simulink model "Full_Charge"  (R2020a)
settings: Solver=VariableStepAuto  StartTime=0.0  StopTime=45*60*60  RelTol=1e-3
values from neighbouring files (symbols this model uses):
  BlySyreON = 1    [sim_starter.m]
  CurrentChargeBlySyre = load    [sim_starter.m]
  CurrentChargeLiLille = load    [sim_starter.m]
  CurrentChargeLiStor = load    [sim_starter.m]
  CurrentChargeNiMH = load    [sim_starter.m]
  CurrentChargeSaltVand = load    [sim_starter.m]
  LiIonLilleON = 1    [sim_starter.m]
  LiIonStorON = 1    [sim_starter.m]
  NiMHON = 1    [sim_starter.m]
  SaltVandON = 1    [sim_starter.m]
  SwitchCurrentBlySyre = 1    [sim_starter.m]
  SwitchCurrentLiLille = 1    [sim_starter.m]
  SwitchCurrentLiStor = 1    [sim_starter.m]
  SwitchCurrentNiMH = 1    [sim_starter.m]
  SwitchCurrentSaltVand = 1    [sim_starter.m]
  VoltageChargeBlySyre = 0    [sim_starter.m]
  VoltageChargeLiLille = load    [sim_starter.m]
  VoltageChargeLiStor = load    [sim_starter.m]
  VoltageChargeNiMH = load    [sim_starter.m]
  VoltageChargeSaltVand = load    [sim_starter.m]
undefined symbols (not defined in the file or in its folder): Hydride, Metal, Nickel
libraries: nesl_utility x37, fl_lib x35, ee_lib x8, powerlib x7, electricdrivelib x1
(part 2 of 2)

== system Full_Charge/Opladning/SaltvandsBatteri ==
  Ah : Constant  Value=45
  Coulomb pr Ah : Constant  Value=3600
  Current Sensor1 : fl_lib/Electrical/Electrical Sensors/Current Sensor
  PS-Simulink Converter : nesl_utility/PS-Simulink Converter  PhysicalDomain=network_engine_domain  SubClassName=ps_output  LeftPortType=input  RightPortType=output  PseudoPeriodic=off  Frequencies=[]  Unit=inherit  AffineConversion=off
  PS-Simulink Converter1 : nesl_utility/PS-Simulink Converter  PhysicalDomain=network_engine_domain  SubClassName=ps_output  LeftPortType=input  RightPortType=output  PseudoPeriodic=off  Frequencies=[]  Unit=inherit  AffineConversion=off
  PS-Simulink Converter2 : nesl_utility/PS-Simulink Converter  PhysicalDomain=network_engine_domain  SubClassName=ps_output  LeftPortType=input  RightPortType=output  PseudoPeriodic=off  Frequencies=[]  Unit=inherit  AffineConversion=off
  Percent SOC : Product  Inputs=*/
  Saltvands : ee_lib/Sources/Battery  Vnom=12 V  R1=0.005 Ohm  prm_AH=2  AH=45 hr*A  V1=10.8 V  AH1=2 hr*A  prm_R2=1  R2=5000 Ohm  prm_dyn=3  Rp1=0.05 Ohm  tau1=700 s  Rp2=0.01 Ohm  tau2=55 s  Rp3=0.005 Ohm  tau3=30 s  Rp4=0.005 Ohm  tau4=30 s  Rp5=0.005 Ohm  tau5=30 s  prm_fade=2  N_fade=5000  AH_fade=36 hr*A  R1_fade=2.02 Ohm  V1_fade=10.35 V  i_specify=off  i_priority=None  i=0 A  i_nominal_specify=off  i_nominal_unit=A  i_nominal_value=1  v_specify=off  v_priority=None  v=0 V  v_nominal_specify=off  v_nominal_unit=V  v_nominal_value=1  charge_specify=on  charge_priority=High  charge=4.5 hr*A  charge_nominal_specify=off  charge_nominal_unit=hr*A  charge_nominal_value=1  num_cycles_specify=off  num_cycles_priority=High  num_cycles=20  num_cycles_nominal_specify=off  num_cycles_nominal_unit=1  num_cycles_nominal_value=1  thermal_mass=30000 J/K  Tmeas=298.15 K  Vnom_T2=12 V  R1_T2=2.2 Ohm  V1_T2=11.4 V  R2_T2=2200 Ohm  Rp1_T2=0.005 Ohm  tau1_T2=30 s  Rp2_T2=0.005 Ohm  tau2_T2=30 s  Rp3_T2=0.005 Ohm  tau3_T2=30 s  Rp4_T2=0.005 Ohm  tau4_T2=30 s  Rp5_T2=0.005 Ohm  tau5_T2=30 s  Tmeas2=273.15 K  temperature_specify=off  temperature_priority=High  temperature=298.15 K  temperature_nominal_specify=off  temperature_nominal_unit=K  temperature_nominal_value=1
      settings: LogSimulationData=on  InternalSimscapePortConfiguration="{\"Bottom\":[],\"Left\":[{\"id\":\"p\",\"label\":\"+\",\"type\":\"foundation.electrical.electrical\"},{\"id\":\"q\",\"label\":\"q\",\"type\":\"output\"}],\"Right\":[{\"id\":\"n\",\"label\":\"-\",\"type\":\"foundation.electrical.electrical\"}],\"Top\":[]}"
  Solver Configuration1 : nesl_utility/Solver Configuration  PhysicalDomain=network_engine_domain  SubClassName=solver  LeftPortType=input  RightPortType=generic  Tones=[]  Harmonics=[]  SimulateNoise=off  Profile=off  UseLocalSampling=off  EnableSwitchedLinearOptims=on  FrequencyDomain=off  UseCCode=off  RelTol=0.001  AbsTol=1e-06  MinStep=1e-09  ToWorkspace=off  RevertToSquareIcSolve=off  NumHomotopyIterations=100  PhasorMode=off  PhasorModeNumHarmonics=1  DoDC=off  ResidualTolerance=1e-09  UseLocalSolver=off  LocalSolverChoice=NE_BACKWARD_EULER_ADVANCER  LocalSolverSampleTime=0.001  DoFixedCost=off  MaxNonlinIter=3  MaxModeIter=2  LinearAlgebra=auto  EquationFormulation=NE_TIME_EF  DelaysMemoryBudget=1024  AutomaticFiltering=on  FilteringTimeConstant=0.001  PartitionStorageMethod=AS_NEEDED  PartitionMemoryBudget=1024  PartitionMethod=ROBUST
  Total Coulomb : Product  Inputs=**
  Voltage Sensor1 : fl_lib/Electrical/Electrical Sensors/Voltage Sensor
  Positiv pin : PMIOPort  Side=Right
  Negativ pin : PMIOPort  Port=2  Side=Right
  voltage : Outport
  current : Outport  Port=2
  SOC : Outport  Port=3
  wires:
  PS-Simulink Converter/1 -> current/1  "Current"
  PS-Simulink Converter1/1 -> voltage/1  "Voltage"
  Total Coulomb/1 -> Percent SOC/2
  PS-Simulink Converter2/1 -> Percent SOC/1  "Current Coulomb"
  Percent SOC/1 -> SOC/1  "State of Charge"
  Ah/1 -> Total Coulomb/1
  Coulomb pr Ah/1 -> Total Coulomb/2
  connections:
  Voltage Sensor1/RConn2 -- Saltvands/RConn1 -- Current Sensor1/RConn2
  Saltvands/LConn1 -- Positiv pin/RConn1 -- Voltage Sensor1/LConn1 -- Solver Configuration1/RConn1
  Current Sensor1/LConn1 -- Negativ pin/RConn1
  Current Sensor1/RConn1 -- PS-Simulink Converter/LConn1
  Voltage Sensor1/RConn1 -- PS-Simulink Converter1/LConn1
  Saltvands/LConn2 -- PS-Simulink Converter2/LConn1

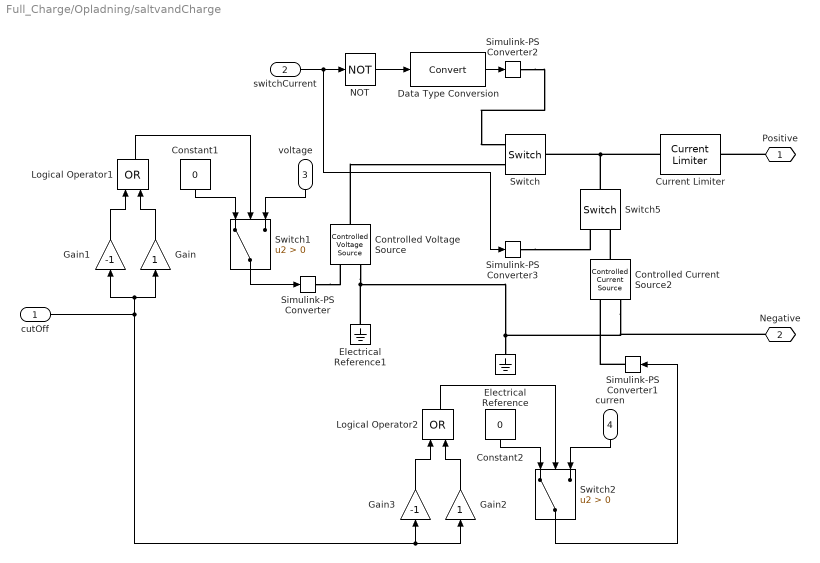
== system Full_Charge/Opladning/saltvandCharge ==
  cutOff : Inport
  switchCurrent : Inport  Port=2
  voltage : Inport  Port=3
  curren : Inport  Port=4
  Constant1 : Constant  Value=0
  Constant2 : Constant  Value=0
  Controlled Current Source2 : fl_lib/Electrical/Electrical Sources/Controlled Current Source
  Controlled Voltage Source : fl_lib/Electrical/Electrical Sources/Controlled Voltage Source
  Current Limiter : ee_lib/Semiconductors & Converters/Current Limiter  iLim=20 A  vLim=0.1 V  gLim=1e-3 1/Ohm  thermal_mass=100 J/K  initial_temperature=298.15 K
      settings: SourceProductBaseCode=PS  InternalSimscapePortConfiguration="{\"Bottom\":[],\"Left\":[{\"id\":\"p\",\"label\":\"+\",\"type\":\"foundation.electrical.electrical\"}],\"Right\":[{\"id\":\"n\",\"label\":\"-\",\"type\":\"foundation.electrical.electrical\"}],\"Top\":[]}"
  Data Type Conversion : DataTypeConversion
  Electrical Reference : fl_lib/Electrical/Electrical Elements/Electrical Reference
  Electrical Reference1 : fl_lib/Electrical/Electrical Elements/Electrical Reference
  Gain : Gain
  Gain1 : Gain  Gain=-1
  Gain2 : Gain
  Gain3 : Gain  Gain=-1
  Logical Operator1 : Logic  Operator=OR  AllPortsSameDT=off  OutDataTypeStr=boolean
  Logical Operator2 : Logic  Operator=OR  AllPortsSameDT=off  OutDataTypeStr=boolean
  NOT : Logic  Operator=NOT  IconShape=distinctive  AllPortsSameDT=off  OutDataTypeStr=boolean
  Simulink-PS Converter : nesl_utility/Simulink-PS Converter  PhysicalDomain=network_engine_domain  SubClassName=ps_input  LeftPortType=input  RightPortType=output  PseudoPeriodic=off  Frequencies=[]  NoiseDistribution=none  NoiseParameters=[]  Unit=V  AffineConversion=off  FilteringAndDerivatives=provide  SimscapeFilterOrder=1  InputFilterTimeConstant=0.001  UdotUserProvided=0
  Simulink-PS Converter1 : nesl_utility/Simulink-PS Converter  PhysicalDomain=network_engine_domain  SubClassName=ps_input  LeftPortType=input  RightPortType=output  PseudoPeriodic=off  Frequencies=[]  NoiseDistribution=none  NoiseParameters=[]  Unit=A  AffineConversion=off  FilteringAndDerivatives=provide  SimscapeFilterOrder=1  InputFilterTimeConstant=0.001  UdotUserProvided=0
  Simulink-PS Converter2 : nesl_utility/Simulink-PS Converter  PhysicalDomain=network_engine_domain  SubClassName=ps_input  LeftPortType=input  RightPortType=output  PseudoPeriodic=off  Frequencies=[]  NoiseDistribution=none  NoiseParameters=[]  Unit=V  AffineConversion=off  FilteringAndDerivatives=provide  SimscapeFilterOrder=1  InputFilterTimeConstant=0.001  UdotUserProvided=0
  Simulink-PS Converter3 : nesl_utility/Simulink-PS Converter  PhysicalDomain=network_engine_domain  SubClassName=ps_input  LeftPortType=input  RightPortType=output  PseudoPeriodic=off  Frequencies=[]  NoiseDistribution=none  NoiseParameters=[]  Unit=V  AffineConversion=off  FilteringAndDerivatives=provide  SimscapeFilterOrder=1  InputFilterTimeConstant=0.001  UdotUserProvided=0
  Switch : fl_lib/Electrical/Electrical Elements/Switch  R_closed=0.01 Ohm  G_open=1e-8 1/Ohm  Threshold=0.5  i_specify=off  i_priority=None  i=0 A  i_nominal_specify=off  i_nominal_unit=A  i_nominal_value=1  v_specify=off  v_priority=None  v=0 V  v_nominal_specify=off  v_nominal_unit=V  v_nominal_value=1
  Switch1 : Switch  Criteria=u2 > Threshold
  Switch2 : Switch  Criteria=u2 > Threshold
  Switch5 : fl_lib/Electrical/Electrical Elements/Switch  R_closed=0.01 Ohm  G_open=1e-8 1/Ohm  Threshold=0.5  i_specify=off  i_priority=None  i=0 A  i_nominal_specify=off  i_nominal_unit=A  i_nominal_value=1  v_specify=off  v_priority=None  v=0 V  v_nominal_specify=off  v_nominal_unit=V  v_nominal_value=1
  Positive : PMIOPort  Side=Left
  Negative : PMIOPort  Port=2  Side=Left
  wires:
  Constant1/1 -> Switch1/1
  Logical Operator1/1 -> Switch1/2
  Gain3/1 -> Logical Operator2/1
  Logical Operator2/1 -> Switch2/2
  Gain/1 -> Logical Operator1/2
  switchCurrent/1 -> Simulink-PS Converter3/1, NOT/1
  NOT/1 -> Data Type Conversion/1
  curren/1 -> Switch2/3
  cutOff/1 -> Gain3/1, Gain2/1, Gain1/1, Gain/1
  Gain2/1 -> Logical Operator2/2
  Gain1/1 -> Logical Operator1/1
  Switch1/1 -> Simulink-PS Converter/1
  voltage/1 -> Switch1/3
  Data Type Conversion/1 -> Simulink-PS Converter2/1
  Constant2/1 -> Switch2/1
  Switch2/1 -> Simulink-PS Converter1/1
  connections:
  Current Limiter/LConn1 -- Switch5/LConn1 -- Switch/LConn1
  Controlled Voltage Source/RConn2 -- Electrical Reference1/LConn1 -- Electrical Reference/LConn1 -- Negative/RConn1 -- Controlled Current Source2/RConn2
  Simulink-PS Converter3/RConn1 -- Switch5/RConn1
  Positive/RConn1 -- Current Limiter/RConn1
  Simulink-PS Converter/RConn1 -- Controlled Voltage Source/RConn1
  Simulink-PS Converter2/RConn1 -- Switch/RConn1
  Simulink-PS Converter1/RConn1 -- Controlled Current Source2/RConn1
  Controlled Voltage Source/LConn1 -- Switch/RConn2
  Controlled Current Source2/LConn1 -- Switch5/RConn2

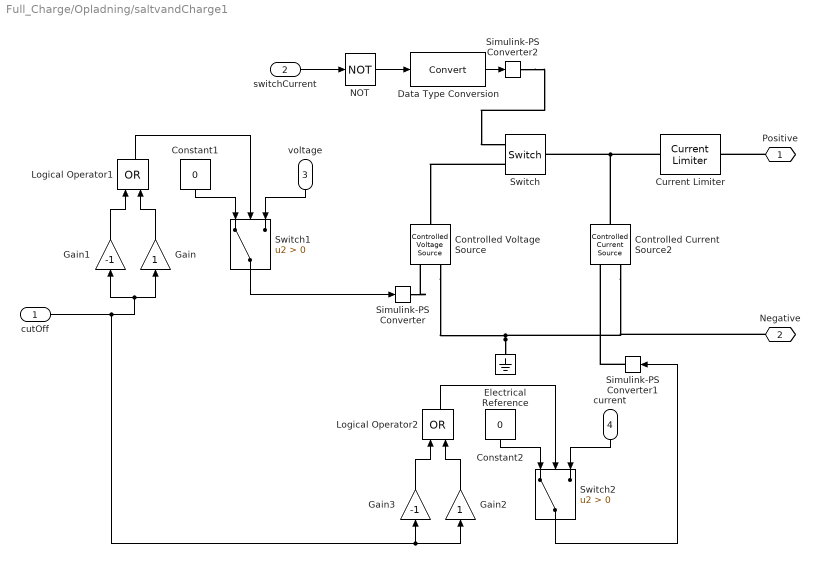
== system Full_Charge/Opladning/saltvandCharge1 ==
  cutOff : Inport
  switchCurrent : Inport  Port=2
  voltage : Inport  Port=3
  current : Inport  Port=4
  Constant1 : Constant  Value=0
  Constant2 : Constant  Value=0
  Controlled Current Source2 : fl_lib/Electrical/Electrical Sources/Controlled Current Source
  Controlled Voltage Source : fl_lib/Electrical/Electrical Sources/Controlled Voltage Source
  Current Limiter : ee_lib/Semiconductors & Converters/Current Limiter  iLim=19 A  vLim=0.1 V  gLim=1e-3 1/Ohm  thermal_mass=100 J/K  initial_temperature=298.15 K
      settings: SourceProductBaseCode=PS  InternalSimscapePortConfiguration="{\"Bottom\":[],\"Left\":[{\"id\":\"p\",\"label\":\"+\",\"type\":\"foundation.electrical.electrical\"}],\"Right\":[{\"id\":\"n\",\"label\":\"-\",\"type\":\"foundation.electrical.electrical\"}],\"Top\":[]}"
  Data Type Conversion : DataTypeConversion
  Electrical Reference : fl_lib/Electrical/Electrical Elements/Electrical Reference
  Gain : Gain
  Gain1 : Gain  Gain=-1
  Gain2 : Gain
  Gain3 : Gain  Gain=-1
  Logical Operator1 : Logic  Operator=OR  AllPortsSameDT=off  OutDataTypeStr=boolean
  Logical Operator2 : Logic  Operator=OR  AllPortsSameDT=off  OutDataTypeStr=boolean
  NOT : Logic  Operator=NOT  IconShape=distinctive  AllPortsSameDT=off  OutDataTypeStr=boolean
  Simulink-PS Converter : nesl_utility/Simulink-PS Converter  PhysicalDomain=network_engine_domain  SubClassName=ps_input  LeftPortType=input  RightPortType=output  PseudoPeriodic=off  Frequencies=[]  NoiseDistribution=none  NoiseParameters=[]  Unit=V  AffineConversion=off  FilteringAndDerivatives=provide  SimscapeFilterOrder=1  InputFilterTimeConstant=0.001  UdotUserProvided=0
  Simulink-PS Converter1 : nesl_utility/Simulink-PS Converter  PhysicalDomain=network_engine_domain  SubClassName=ps_input  LeftPortType=input  RightPortType=output  PseudoPeriodic=off  Frequencies=[]  NoiseDistribution=none  NoiseParameters=[]  Unit=A  AffineConversion=off  FilteringAndDerivatives=provide  SimscapeFilterOrder=1  InputFilterTimeConstant=0.001  UdotUserProvided=0
  Simulink-PS Converter2 : nesl_utility/Simulink-PS Converter  PhysicalDomain=network_engine_domain  SubClassName=ps_input  LeftPortType=input  RightPortType=output  PseudoPeriodic=off  Frequencies=[]  NoiseDistribution=none  NoiseParameters=[]  Unit=V  AffineConversion=off  FilteringAndDerivatives=provide  SimscapeFilterOrder=1  InputFilterTimeConstant=0.001  UdotUserProvided=0
  Switch : fl_lib/Electrical/Electrical Elements/Switch  R_closed=0.01 Ohm  G_open=1e-8 1/Ohm  Threshold=0.5  i_specify=off  i_priority=None  i=0 A  i_nominal_specify=off  i_nominal_unit=A  i_nominal_value=1  v_specify=off  v_priority=None  v=0 V  v_nominal_specify=off  v_nominal_unit=V  v_nominal_value=1
  Switch1 : Switch  Criteria=u2 > Threshold
  Switch2 : Switch  Criteria=u2 > Threshold
  Positive : PMIOPort  Side=Left
  Negative : PMIOPort  Port=2  Side=Left
  wires:
  Data Type Conversion/1 -> Simulink-PS Converter2/1
  NOT/1 -> Data Type Conversion/1
  switchCurrent/1 -> NOT/1
  voltage/1 -> Switch1/3
  Constant1/1 -> Switch1/1
  Logical Operator1/1 -> Switch1/2
  Gain1/1 -> Logical Operator1/1
  Switch1/1 -> Simulink-PS Converter/1
  Gain/1 -> Logical Operator1/2
  cutOff/1 -> Gain3/1, Gain2/1, Gain1/1, Gain/1
  Gain2/1 -> Logical Operator2/2
  current/1 -> Switch2/3
  Gain3/1 -> Logical Operator2/1
  Constant2/1 -> Switch2/1
  Logical Operator2/1 -> Switch2/2
  Switch2/1 -> Simulink-PS Converter1/1
  connections:
  Positive/RConn1 -- Current Limiter/RConn1
  Switch/RConn2 -- Controlled Voltage Source/LConn1
  Simulink-PS Converter1/RConn1 -- Controlled Current Source2/RConn1
  Simulink-PS Converter2/RConn1 -- Switch/RConn1
  Simulink-PS Converter/RConn1 -- Controlled Voltage Source/RConn1
  Electrical Reference/LConn1 -- Controlled Voltage Source/RConn2 -- Controlled Current Source2/RConn2 -- Negative/RConn1
  Current Limiter/LConn1 -- Controlled Current Source2/LConn1 -- Switch/LConn1

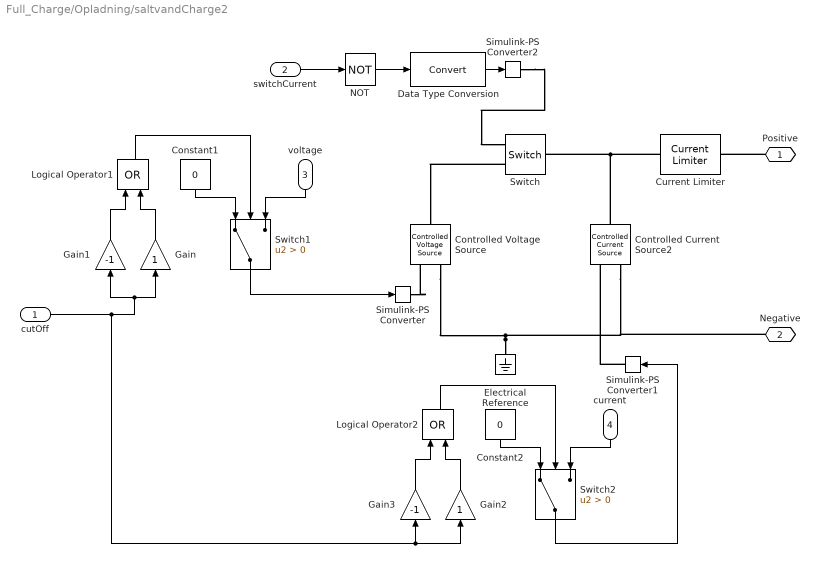
== system Full_Charge/Opladning/saltvandCharge2 ==
  cutOff : Inport
  switchCurrent : Inport  Port=2
  voltage : Inport  Port=3
  current : Inport  Port=4
  Constant1 : Constant  Value=0
  Constant2 : Constant  Value=0
  Controlled Current Source2 : fl_lib/Electrical/Electrical Sources/Controlled Current Source
  Controlled Voltage Source : fl_lib/Electrical/Electrical Sources/Controlled Voltage Source
  Current Limiter : ee_lib/Semiconductors & Converters/Current Limiter  iLim=19 A  vLim=0.1 V  gLim=1e-3 1/Ohm  thermal_mass=100 J/K  initial_temperature=298.15 K
      settings: SourceProductBaseCode=PS  InternalSimscapePortConfiguration="{\"Bottom\":[],\"Left\":[{\"id\":\"p\",\"label\":\"+\",\"type\":\"foundation.electrical.electrical\"}],\"Right\":[{\"id\":\"n\",\"label\":\"-\",\"type\":\"foundation.electrical.electrical\"}],\"Top\":[]}"
  Data Type Conversion : DataTypeConversion
  Electrical Reference : fl_lib/Electrical/Electrical Elements/Electrical Reference
  Gain : Gain
  Gain1 : Gain  Gain=-1
  Gain2 : Gain
  Gain3 : Gain  Gain=-1
  Logical Operator1 : Logic  Operator=OR  AllPortsSameDT=off  OutDataTypeStr=boolean
  Logical Operator2 : Logic  Operator=OR  AllPortsSameDT=off  OutDataTypeStr=boolean
  NOT : Logic  Operator=NOT  IconShape=distinctive  AllPortsSameDT=off  OutDataTypeStr=boolean
  Simulink-PS Converter : nesl_utility/Simulink-PS Converter  PhysicalDomain=network_engine_domain  SubClassName=ps_input  LeftPortType=input  RightPortType=output  PseudoPeriodic=off  Frequencies=[]  NoiseDistribution=none  NoiseParameters=[]  Unit=V  AffineConversion=off  FilteringAndDerivatives=provide  SimscapeFilterOrder=1  InputFilterTimeConstant=0.001  UdotUserProvided=0
  Simulink-PS Converter1 : nesl_utility/Simulink-PS Converter  PhysicalDomain=network_engine_domain  SubClassName=ps_input  LeftPortType=input  RightPortType=output  PseudoPeriodic=off  Frequencies=[]  NoiseDistribution=none  NoiseParameters=[]  Unit=A  AffineConversion=off  FilteringAndDerivatives=provide  SimscapeFilterOrder=1  InputFilterTimeConstant=0.001  UdotUserProvided=0
  Simulink-PS Converter2 : nesl_utility/Simulink-PS Converter  PhysicalDomain=network_engine_domain  SubClassName=ps_input  LeftPortType=input  RightPortType=output  PseudoPeriodic=off  Frequencies=[]  NoiseDistribution=none  NoiseParameters=[]  Unit=V  AffineConversion=off  FilteringAndDerivatives=provide  SimscapeFilterOrder=1  InputFilterTimeConstant=0.001  UdotUserProvided=0
  Switch : fl_lib/Electrical/Electrical Elements/Switch  R_closed=0.01 Ohm  G_open=1e-8 1/Ohm  Threshold=0.5  i_specify=off  i_priority=None  i=0 A  i_nominal_specify=off  i_nominal_unit=A  i_nominal_value=1  v_specify=off  v_priority=None  v=0 V  v_nominal_specify=off  v_nominal_unit=V  v_nominal_value=1
  Switch1 : Switch  Criteria=u2 > Threshold
  Switch2 : Switch  Criteria=u2 > Threshold
  Positive : PMIOPort  Side=Left
  Negative : PMIOPort  Port=2  Side=Left
  wires:
  Data Type Conversion/1 -> Simulink-PS Converter2/1
  NOT/1 -> Data Type Conversion/1
  switchCurrent/1 -> NOT/1
  voltage/1 -> Switch1/3
  Constant1/1 -> Switch1/1
  Logical Operator1/1 -> Switch1/2
  Gain1/1 -> Logical Operator1/1
  Switch1/1 -> Simulink-PS Converter/1
  Gain/1 -> Logical Operator1/2
  cutOff/1 -> Gain3/1, Gain2/1, Gain1/1, Gain/1
  Gain2/1 -> Logical Operator2/2
  current/1 -> Switch2/3
  Gain3/1 -> Logical Operator2/1
  Constant2/1 -> Switch2/1
  Logical Operator2/1 -> Switch2/2
  Switch2/1 -> Simulink-PS Converter1/1
  connections:
  Positive/RConn1 -- Current Limiter/RConn1
  Switch/RConn2 -- Controlled Voltage Source/LConn1
  Simulink-PS Converter1/RConn1 -- Controlled Current Source2/RConn1
  Simulink-PS Converter2/RConn1 -- Switch/RConn1
  Simulink-PS Converter/RConn1 -- Controlled Voltage Source/RConn1
  Electrical Reference/LConn1 -- Controlled Voltage Source/RConn2 -- Controlled Current Source2/RConn2 -- Negative/RConn1
  Current Limiter/LConn1 -- Controlled Current Source2/LConn1 -- Switch/LConn1

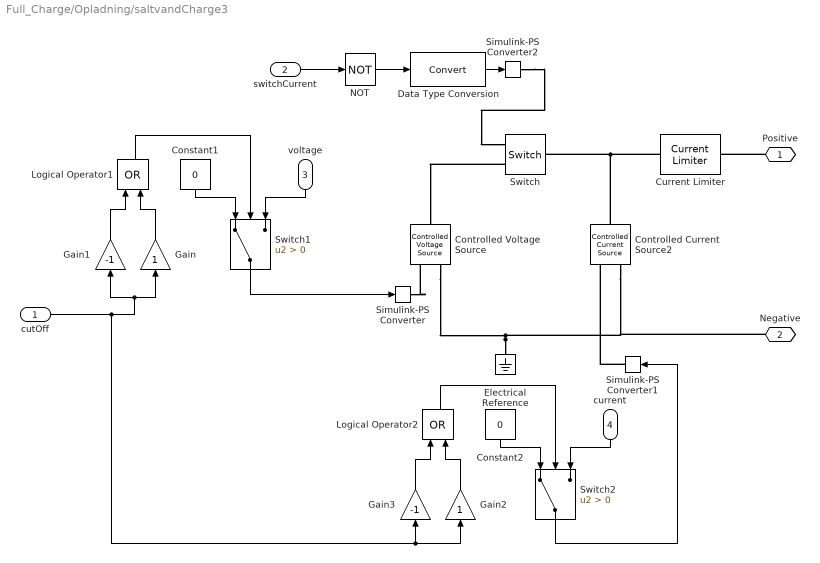
== system Full_Charge/Opladning/saltvandCharge3 ==
  cutOff : Inport
  switchCurrent : Inport  Port=2
  voltage : Inport  Port=3
  current : Inport  Port=4
  Constant1 : Constant  Value=0
  Constant2 : Constant  Value=0
  Controlled Current Source2 : fl_lib/Electrical/Electrical Sources/Controlled Current Source
  Controlled Voltage Source : fl_lib/Electrical/Electrical Sources/Controlled Voltage Source
  Current Limiter : ee_lib/Semiconductors & Converters/Current Limiter  iLim=19 A  vLim=0.1 V  gLim=1e-3 1/Ohm  thermal_mass=100 J/K  initial_temperature=298.15 K
      settings: SourceProductBaseCode=PS  InternalSimscapePortConfiguration="{\"Bottom\":[],\"Left\":[{\"id\":\"p\",\"label\":\"+\",\"type\":\"foundation.electrical.electrical\"}],\"Right\":[{\"id\":\"n\",\"label\":\"-\",\"type\":\"foundation.electrical.electrical\"}],\"Top\":[]}"
  Data Type Conversion : DataTypeConversion
  Electrical Reference : fl_lib/Electrical/Electrical Elements/Electrical Reference
  Gain : Gain
  Gain1 : Gain  Gain=-1
  Gain2 : Gain
  Gain3 : Gain  Gain=-1
  Logical Operator1 : Logic  Operator=OR  AllPortsSameDT=off  OutDataTypeStr=boolean
  Logical Operator2 : Logic  Operator=OR  AllPortsSameDT=off  OutDataTypeStr=boolean
  NOT : Logic  Operator=NOT  IconShape=distinctive  AllPortsSameDT=off  OutDataTypeStr=boolean
  Simulink-PS Converter : nesl_utility/Simulink-PS Converter  PhysicalDomain=network_engine_domain  SubClassName=ps_input  LeftPortType=input  RightPortType=output  PseudoPeriodic=off  Frequencies=[]  NoiseDistribution=none  NoiseParameters=[]  Unit=V  AffineConversion=off  FilteringAndDerivatives=provide  SimscapeFilterOrder=1  InputFilterTimeConstant=0.001  UdotUserProvided=0
  Simulink-PS Converter1 : nesl_utility/Simulink-PS Converter  PhysicalDomain=network_engine_domain  SubClassName=ps_input  LeftPortType=input  RightPortType=output  PseudoPeriodic=off  Frequencies=[]  NoiseDistribution=none  NoiseParameters=[]  Unit=A  AffineConversion=off  FilteringAndDerivatives=provide  SimscapeFilterOrder=1  InputFilterTimeConstant=0.001  UdotUserProvided=0
  Simulink-PS Converter2 : nesl_utility/Simulink-PS Converter  PhysicalDomain=network_engine_domain  SubClassName=ps_input  LeftPortType=input  RightPortType=output  PseudoPeriodic=off  Frequencies=[]  NoiseDistribution=none  NoiseParameters=[]  Unit=V  AffineConversion=off  FilteringAndDerivatives=provide  SimscapeFilterOrder=1  InputFilterTimeConstant=0.001  UdotUserProvided=0
  Switch : fl_lib/Electrical/Electrical Elements/Switch  R_closed=0.01 Ohm  G_open=1e-8 1/Ohm  Threshold=0.5  i_specify=off  i_priority=None  i=0 A  i_nominal_specify=off  i_nominal_unit=A  i_nominal_value=1  v_specify=off  v_priority=None  v=0 V  v_nominal_specify=off  v_nominal_unit=V  v_nominal_value=1
  Switch1 : Switch  Criteria=u2 > Threshold
  Switch2 : Switch  Criteria=u2 > Threshold
  Positive : PMIOPort  Side=Left
  Negative : PMIOPort  Port=2  Side=Left
  wires:
  Data Type Conversion/1 -> Simulink-PS Converter2/1
  NOT/1 -> Data Type Conversion/1
  switchCurrent/1 -> NOT/1
  voltage/1 -> Switch1/3
  Constant1/1 -> Switch1/1
  Logical Operator1/1 -> Switch1/2
  Gain1/1 -> Logical Operator1/1
  Switch1/1 -> Simulink-PS Converter/1
  Gain/1 -> Logical Operator1/2
  cutOff/1 -> Gain3/1, Gain2/1, Gain1/1, Gain/1
  Gain2/1 -> Logical Operator2/2
  current/1 -> Switch2/3
  Gain3/1 -> Logical Operator2/1
  Constant2/1 -> Switch2/1
  Logical Operator2/1 -> Switch2/2
  Switch2/1 -> Simulink-PS Converter1/1
  connections:
  Positive/RConn1 -- Current Limiter/RConn1
  Switch/RConn2 -- Controlled Voltage Source/LConn1
  Simulink-PS Converter1/RConn1 -- Controlled Current Source2/RConn1
  Simulink-PS Converter2/RConn1 -- Switch/RConn1
  Simulink-PS Converter/RConn1 -- Controlled Voltage Source/RConn1
  Electrical Reference/LConn1 -- Controlled Voltage Source/RConn2 -- Controlled Current Source2/RConn2 -- Negative/RConn1
  Current Limiter/LConn1 -- Controlled Current Source2/LConn1 -- Switch/LConn1

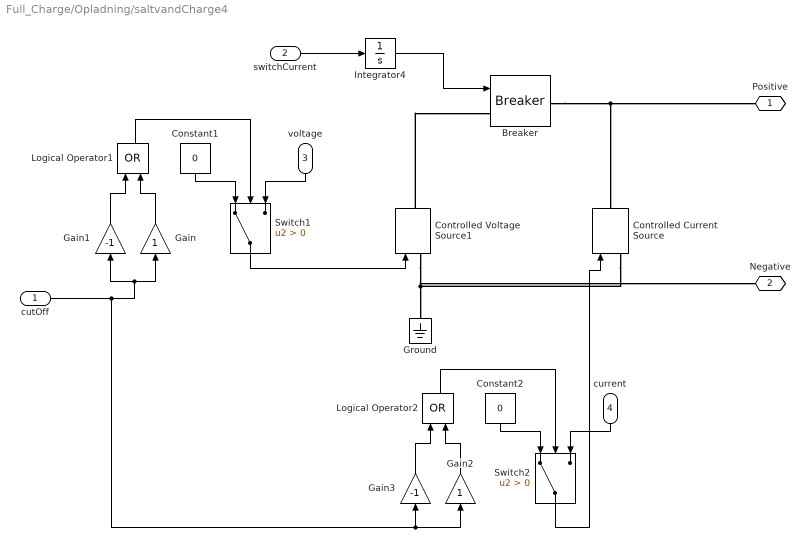
== system Full_Charge/Opladning/saltvandCharge4 ==
  cutOff : Inport
  switchCurrent : Inport  Port=2
  voltage : Inport  Port=3
  current : Inport  Port=4
  Breaker : powerlib/Elements/Breaker  InitialState=0  SwitchingTimes="[1/60  5/60]"  External=on  BreakerResistance=0.01  SnubberResistance=1e6  SnubberCapacitance=inf  Measurements=None  MoreParameters=on  NoBreakLoop=off
  Constant1 : Constant  Value=0
  Constant2 : Constant  Value=0
  Controlled Current Source : powerlib/Electrical Sources/Controlled Current Source  Initialize=on  Source_Type=AC  Amplitude=0  Phase=0  Frequency=0  Measurements=None
  Controlled Voltage Source1 : powerlib/Electrical Sources/Controlled Voltage Source  Initialize=on  Source_Type=AC  Amplitude=0  Phase=0  Frequency=0  Measurements=None
  Gain : Gain
  Gain1 : Gain  Gain=-1
  Gain2 : Gain
  Gain3 : Gain  Gain=-1
  Ground : powerlib/Elements/Ground  LConnTagsString=a
  Integrator4 : Integrator
  Logical Operator1 : Logic  Operator=OR  AllPortsSameDT=off  OutDataTypeStr=boolean
  Logical Operator2 : Logic  Operator=OR  AllPortsSameDT=off  OutDataTypeStr=boolean
  Switch1 : Switch  Criteria=u2 > Threshold
  Switch2 : Switch  Criteria=u2 > Threshold
  Positive : PMIOPort  Side=Left
  Negative : PMIOPort  Port=2  Side=Left
  wires:
  switchCurrent/1 -> Integrator4/1
  voltage/1 -> Switch1/3
  Constant1/1 -> Switch1/1
  Logical Operator1/1 -> Switch1/2
  Gain1/1 -> Logical Operator1/1
  Gain/1 -> Logical Operator1/2
  cutOff/1 -> Gain3/1, Gain2/1, Gain1/1, Gain/1
  Gain2/1 -> Logical Operator2/2
  current/1 -> Switch2/3
  Gain3/1 -> Logical Operator2/1
  Constant2/1 -> Switch2/1
  Logical Operator2/1 -> Switch2/2
  Integrator4/1 -> Breaker/1
  Switch1/1 -> Controlled Voltage Source1/1
  Switch2/1 -> Controlled Current Source/1
  connections:
  Controlled Voltage Source1/RConn1 -- Breaker/LConn1
  Controlled Voltage Source1/LConn1 -- Controlled Current Source/LConn1 -- Negative/RConn1 -- Ground/LConn1
  Breaker/RConn1 -- Positive/RConn1 -- Controlled Current Source/RConn1

== stateflow chart Full_Charge/Opladning/BMS Saltvand /BMS kontrol ==
  state Idle
    %I dette stadie er vores BMS idle, da der hverken sker opladning eller afladning af vores batteri.
    entry:
    cutOff = 0;
  state Charging
    during:
    discharging = 0;
    charging = 1;
    state dischargingLevel
      entry:
      cutOff = 0;
    state currentLevel
      entry:
      cutOff = 1;
    state voltageLevel
      entry:
      cutOff = 1;
    (default) -> Charging.dischargingLevel
    Charging.dischargingLevel -> Charging.currentLevel [order 2] : [currentLevel >= currentUpperLimitCharge | SOC >= 1]{cutOff =  1;}
    Charging.currentLevel -> Charging.dischargingLevel : [currentLevel <= currentUpperLimitCharge]{cutOff = 0;}
    Charging.dischargingLevel -> Charging.voltageLevel [order 1] : [voltageLevel >= voltageUpperLimit | SOC >= 1]{cutOff = 1;}
  state Discharge
    entry:
    discharging = 1;
    charging = 0;
    state dischargingLevel
    state currentLevel
    state voltageLevel
    (default) -> Discharge.dischargingLevel
    Discharge.dischargingLevel -> Discharge.currentLevel [order 2] : [currentLevel >= currentUpperLimit | SOC <= 0.05]{cutOff =  1;}
    Discharge.currentLevel -> Discharge.dischargingLevel : [currentLevel <= currentUpperLimit]{cutOff = 0;}
    Discharge.dischargingLevel -> Discharge.voltageLevel [order 1] : [voltageLevel <= voltageLowerLimit | SOC <= 0.05]{cutOff = 1;}
  (default) -> Idle
  Discharge -> Idle [order 2] : [currentLevel == 0]
  Idle -> Discharge [order 1] : [currentLevel >= 0]
  Charging -> Idle [order 2] : [currentLevel == 0]
  Idle -> Charging [order 2] : [currentLevel <= 0 ]
  Discharge -> Charging [order 1] : [currentLevel <= 0 ]
  Charging -> Discharge [order 1] : [currentLevel >= 0]
  data: currentLevel input; voltageLevel input; discharging local; charging local; cutOff output; currentUpperLimit local =20; SOC input; voltageLowerLimit local =9.0; voltageUpperLimit local =20; currentUpperLimitCharge local =20

== stateflow chart Full_Charge/Opladning/BMS Li ion Stor/BMS kontrol ==
  state Idle
    %I dette stadie er vores BMS idle, da der hverken sker opladning eller afladning af vores batteri.
  state Charging
    during:
    discharging = 0;
    charging = 1;
    state dischargingLevel
      entry:
      cutOff = 0;
    state currentLevel
      entry:
      cutOff = 1;
    state voltageLevel
      entry:
      cutOff = 1;
    (default) -> Charging.dischargingLevel
    Charging.dischargingLevel -> Charging.currentLevel [order 2] : [currentLevel >= currentUpperLimitCharge | SOC >= 1]{cutOff =  1;}
    Charging.currentLevel -> Charging.dischargingLevel : [currentLevel <= currentUpperLimitCharge]{cutOff = 0;}
    Charging.dischargingLevel -> Charging.voltageLevel [order 1] : [voltageLevel >= voltageUpperLimit | SOC >= 1]{cutOff = 1;}
  state Discharge
    entry:
    discharging = 1;
    charging = 0;
    state dischargingLevel
    state currentLevel
    state voltageLevel
    (default) -> Discharge.dischargingLevel
    Discharge.dischargingLevel -> Discharge.currentLevel [order 2] : [currentLevel >= currentUpperLimit | SOC <= 0.05]{cutOff =  1;}
    Discharge.currentLevel -> Discharge.dischargingLevel : [currentLevel <= currentUpperLimit]{cutOff = 0;}
    Discharge.dischargingLevel -> Discharge.voltageLevel [order 1] : [voltageLevel <= voltageLowerLimit | SOC <= 0.05]{cutOff = 1;}
  (default) -> Idle
  Discharge -> Idle [order 2] : [currentLevel == 0]
  Idle -> Discharge [order 1] : [currentLevel >= 0]
  Charging -> Idle [order 2] : [currentLevel == 0]
  Idle -> Charging [order 2] : [currentLevel <= 0 ]
  Discharge -> Charging [order 1] : [currentLevel <= 0 ]
  Charging -> Discharge [order 1] : [currentLevel >= 0]
  data: currentLevel input; voltageLevel input; discharging local; charging local; cutOff output; currentUpperLimit local =20; SOC input; voltageLowerLimit local =9.0; voltageUpperLimit local =20; currentUpperLimitCharge local =20

== stateflow chart Full_Charge/Opladning/BMS Li Ion Lille/BMS kontrol ==
  state Idle
    %I dette stadie er vores BMS idle, da der hverken sker opladning eller afladning af vores batteri.
  state Charging
    during:
    discharging = 0;
    charging = 1;
    state dischargingLevel
      entry:
      cutOff = 0;
    state currentLevel
      entry:
      cutOff = 1;
    state voltageLevel
      entry:
      cutOff = 1;
    (default) -> Charging.dischargingLevel
    Charging.dischargingLevel -> Charging.currentLevel [order 2] : [currentLevel >= currentUpperLimitCharge | SOC >= 1]{cutOff =  1;}
    Charging.currentLevel -> Charging.dischargingLevel : [currentLevel <= currentUpperLimitCharge]{cutOff = 0;}
    Charging.dischargingLevel -> Charging.voltageLevel [order 1] : [voltageLevel >= voltageUpperLimit | SOC >= 1]{cutOff = 1;}
  state Discharge
    entry:
    discharging = 1;
    charging = 0;
    state dischargingLevel
    state currentLevel
    state voltageLevel
    (default) -> Discharge.dischargingLevel
    Discharge.dischargingLevel -> Discharge.currentLevel [order 2] : [currentLevel >= currentUpperLimit | SOC <= 0.05]{cutOff =  1;}
    Discharge.currentLevel -> Discharge.dischargingLevel : [currentLevel <= currentUpperLimit]{cutOff = 0;}
    Discharge.dischargingLevel -> Discharge.voltageLevel [order 1] : [voltageLevel <= voltageLowerLimit | SOC <= 0.05]{cutOff = 1;}
  (default) -> Idle
  Discharge -> Idle [order 2] : [currentLevel == 0]
  Idle -> Discharge [order 1] : [currentLevel >= 0]
  Charging -> Idle [order 2] : [currentLevel == 0]
  Idle -> Charging [order 2] : [currentLevel <= 0 ]
  Discharge -> Charging [order 1] : [currentLevel <= 0 ]
  Charging -> Discharge [order 1] : [currentLevel >= 0]
  data: currentLevel input; voltageLevel input; discharging local; charging local; cutOff output; currentUpperLimit local =0.52; SOC input; voltageLowerLimit local =3; voltageUpperLimit local =5; currentUpperLimitCharge local =0.52

== stateflow chart Full_Charge/Opladning/BMS NiMH/BMS kontrol ==
  state Idle
    %I dette stadie er vores BMS idle, da der hverken sker opladning eller afladning af vores batteri.
  state Charging
    during:
    discharging = 0;
    charging = 1;
    state dischargingLevel
      entry:
      cutOff = 0;
    state currentLevel
      entry:
      cutOff = 1;
    state voltageLevel
      entry:
      cutOff = 1;
    (default) -> Charging.dischargingLevel
    Charging.dischargingLevel -> Charging.currentLevel [order 2] : [currentLevel >= currentUpperLimitCharge | SOC >= 1]{cutOff =  1;}
    Charging.currentLevel -> Charging.dischargingLevel : [currentLevel <= currentUpperLimitCharge]{cutOff = 0;}
    Charging.dischargingLevel -> Charging.voltageLevel [order 1] : [voltageLevel >= voltageUpperLimit | SOC >= 1]{cutOff = 1;}
  state Discharge
    entry:
    discharging = 1;
    charging = 0;
    state dischargingLevel
    state currentLevel
    state voltageLevel
    (default) -> Discharge.dischargingLevel
    Discharge.dischargingLevel -> Discharge.currentLevel [order 2] : [currentLevel >= currentUpperLimit | SOC <=0.05]{cutOff =  1;}
    Discharge.currentLevel -> Discharge.dischargingLevel : [currentLevel <= currentUpperLimit]{cutOff = 0;}
    Discharge.dischargingLevel -> Discharge.voltageLevel [order 1] : [voltageLevel <= voltageLowerLimit | SOC <= 0.05]{cutOff = 1;}
  (default) -> Idle
  Discharge -> Idle [order 2] : [currentLevel == 0]
  Idle -> Discharge [order 1] : [currentLevel >= 0]
  Charging -> Idle [order 2] : [currentLevel == 0]
  Idle -> Charging [order 2] : [currentLevel <= 0 ]
  Discharge -> Charging [order 1] : [currentLevel <= 0 ]
  Charging -> Discharge [order 1] : [currentLevel >= 0]
  data: currentLevel input; voltageLevel input; discharging local; charging local; cutOff output; currentUpperLimit local =1.2; SOC input; voltageLowerLimit local =1; voltageUpperLimit local =2.43; currentUpperLimitCharge local =1

== stateflow chart Full_Charge/Opladning/BMS BlySyre/BMS kontrol ==
  state Idle
    %I dette stadie er vores BMS idle, da der hverken sker opladning eller afladning af vores batteri.
  state Charging
    during:
    discharging = 0;
    charging = 1;
    state dischargingLevel
      entry:
      cutOff = 0;
    state currentLevel
      entry:
      cutOff = 1;
    state voltageLevel
      entry:
      cutOff = 1;
    (default) -> Charging.dischargingLevel
    Charging.dischargingLevel -> Charging.currentLevel [order 2] : [currentLevel >= currentUpperLimitCharge | SOC >= 1]{cutOff =  1;}
    Charging.currentLevel -> Charging.dischargingLevel : [currentLevel <= currentUpperLimitCharge]{cutOff = 0;}
    Charging.dischargingLevel -> Charging.voltageLevel [order 1] : [voltageLevel >= voltageUpperLimit | SOC >= 1]{cutOff = 1;}
  state Discharge
    entry:
    discharging = 1;
    charging = 0;
    state dischargingLevel
    state currentLevel
    state voltageLevel
    (default) -> Discharge.dischargingLevel
    Discharge.dischargingLevel -> Discharge.currentLevel [order 2] : [currentLevel >= currentUpperLimit | SOC <= 0.05]{cutOff =  1;}
    Discharge.currentLevel -> Discharge.dischargingLevel : [currentLevel <= currentUpperLimit]{cutOff = 0;}
    Discharge.dischargingLevel -> Discharge.voltageLevel [order 1] : [voltageLevel <= voltageLowerLimit | SOC <= 0.05]{cutOff = 1;}
  (default) -> Idle
  Discharge -> Idle [order 2] : [currentLevel == 0]
  Idle -> Discharge [order 1] : [currentLevel >= 0]
  Charging -> Idle [order 2] : [currentLevel == 0]
  Idle -> Charging [order 2] : [currentLevel <= 0 ]
  Discharge -> Charging [order 1] : [currentLevel <= 0 ]
  Charging -> Discharge [order 1] : [currentLevel >= 0]
  data: currentLevel input; voltageLevel input; discharging local; charging local; cutOff output; currentUpperLimit local =20; SOC input; voltageLowerLimit local =10; voltageUpperLimit local =20; currentUpperLimitCharge local =20
